simulink model "group_2_4081_4102_4209_"  (R2020a)
settings: Solver=ode23t  StartTime=0.0  StopTime=10  RelTol=1e-3
undefined symbols (not defined in the file): Acid, Lead, sigbuilder_block
libraries: powerlib x49, simulink x7, powerlib_meascontrol x5, electricdrivelib x1, re_lib x1
settings Model: Creator=ASUS  LastModifiedBy=Mushrif
settings DataIOCC: SaveOutput=off  SaveState=on  SignalLogging=off  DSMLogging=off  ReturnWorkspaceOutputs=off  LoggingToFile=on
settings DebuggingCC: UnconnectedInputMsg=none  UnconnectedOutputMsg=none  UnconnectedLineMsg=none  SFMachineParentedDataDiag=error
settings ModelReferenceCC: EnableRefExpFcnMdlSchedulingChecks=off
settings RTWCC: Description=Generic Real-Time Target

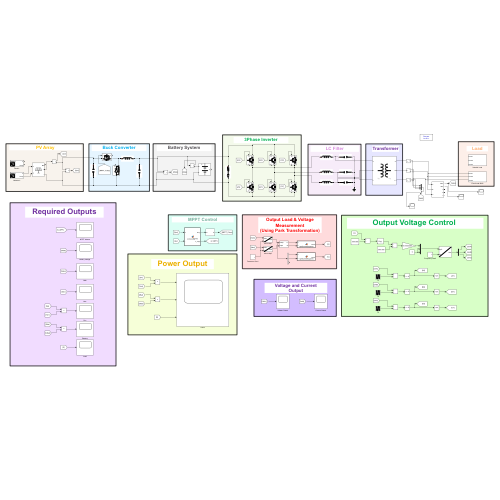
[thumbnail: Simulink's stored preview of the top-level diagram]
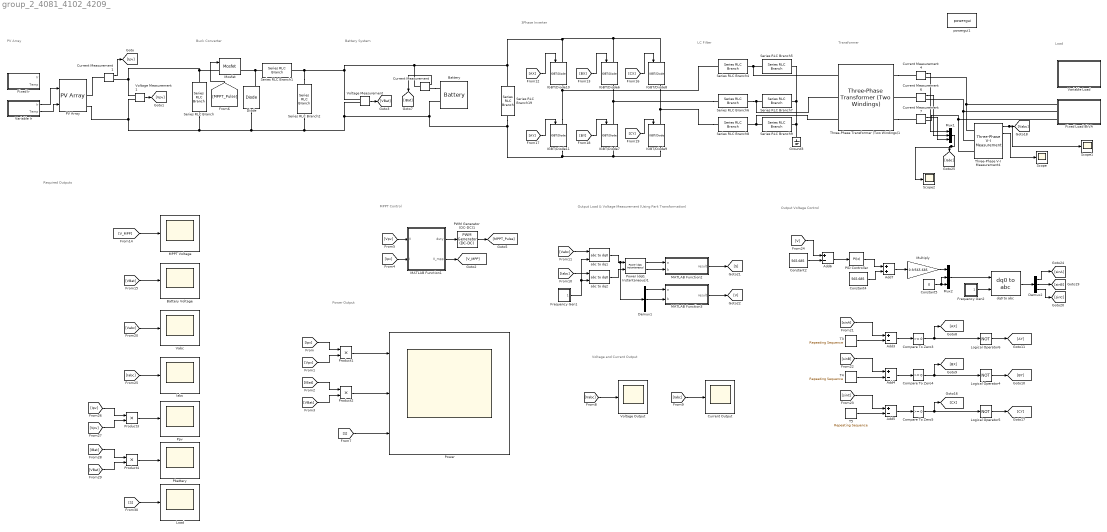
== system group_2_4081_4102_4209_ ==
  note: PV Array
  note: Buck Converter
  note: Battery System
  note: 3Phase Inverter
  note: LC Filter
  note: Load
  note: Transformer
  note: MPPT Control
  note: Power Output
  note: Output Load & Voltage Measurement
      | (Using Park Transformation)
  note: Output Voltage Control
  note: Voltage and Current
      | Output
  note: Required Outputs
  Add{3..6} (4 alike) : Sum  Inputs=+-
  Add7 : Sum
  Battery : electricdrivelib/Extra Sources/Battery  BatType=Lead-Acid  ShowTempParam=off  ThermalPreset=no  ShowAgeParam=off  NomV=48  NomQ=833.33  SOC=50  Batt_Tr=1  PresetModel=off  MaxQ=5.4  MinV=36  FullV=48  Dis_rate=2.3478  R=0.013333  Normal_OP=4.8835  expZone="[48     0.2653]"  current=[6.5 13 32.5]  Units=Time  Tci=20  NomT=20  T2=-30  MaxQ2=4.8  FullV2=7.1  Normal_OP2=5.655  expZone2="[6.58           1]"  Rca=0.6  ti=2000  Dp=0  Neq0=0  Tsim=1e6  Ta1=25  Qeol=5.4*0.9  Reol=0.013333*1.2  Char_age=[2.3478, 3]  Dis_age=[2.3478, 10]  N1=1500  N2=10500  N3=1000  N4=1400  Ta2=45  N5=950
  Battery Voltage : Scope
  Compare To Zero3 : simulink/Logic and Bit Operations/Compare To Zero  relop=>=  OutDataTypeStr=boolean
  Compare To Zero4 : simulink/Logic and Bit Operations/Compare To Zero  relop=>=  OutDataTypeStr=boolean
  Compare To Zero5 : simulink/Logic and Bit Operations/Compare To Zero  relop=>=  OutDataTypeStr=boolean
  Constant2 : Constant  Value=565.685
  Constant4 : Constant  Value=565.685
  Constant5 : Constant  Value=0
  Current Measurement{,1,4,6..7} (5 alike) : powerlib/Measurements/Current Measurement  PhasorSimulation=off  OutputType=Complex  PSBequivalent=0
  Current Output : Scope
  Demux1 : Demux  Outputs=3
  Demux2 : Demux  Outputs=3
  Diode : powerlib/Power Electronics/Diode  Ron=0.001  Lon=0  Vf=0.8  IC=0  UseSnubber=0  Rs=500  Cs=250e-9  Measurements=on
  Fixed Ir : Subsystem  Tag=STV Subsys  LoadFcn=sigbuilder_block('load');  StartFcn=sigbuilder_block('start');  StopFcn=sigbuilder_block('stop');  ClipboardFcn=sigbuilder_block('clipboard');  mask(Sigbuilder block){tuvar=[0:10]}
      mask help: Simulink:masks:SigbuilderBlock_MD
      mask init:
      | if ~strcmp(get_param(bdroot(gcbh),'SimulationStatus'),'stopped') tuvar = sigbuilder_block('maskInit'); end
      settings: CopyFcn=sigbuilder_block('copy');  DeleteFcn=sigbuilder_block('delete');  ModelCloseFcn=sigbuilder_block('modelClose');  PreSaveFcn=sigbuilder_block('preSave');  PauseFcn=sigbuilder_block('pause');  ContinueFcn=sigbuilder_block('continue');  NameChangeFcn=sigbuilder_block('namechange');  OpenFcn=sigbuilder_block('open',[437.6 182.4 550.4 400.2 ]);  CloseFcn=sigbuilder_block('close');
      mask Display: plot(0, 0, 100, 100,[2, 2, 32, 32, 2], [68, 8, 8, 68, 68],[32, 2], [38, 38], [32, 19, 2],[53, 60, 44], [32, 17, 17, 2],[16, 16, 31, 31]);txt = getActiveGroup(gcbh);text(2, 100, txt,'verticalAlignment', 'top');
  Fixed Load 8kVA : Subsystem
  Frequency Gen1 : Subsystem
  Frequency Gen2 : Subsystem
  Ground3 : powerlib/Elements/Ground  LConnTagsString=a
  IGBT/Diode{6..11} (6 alike) : powerlib/Power Electronics/IGBT//Diode  Ron=1e-3  Rs=1e5  Cs=inf  Measurements=on
  Iabc : Scope
  Load : Scope
  Logical Operator4 : Logic  Operator=NOT  AllPortsSameDT=off  OutDataTypeStr=boolean
  Logical Operator5 : Logic  Operator=NOT  AllPortsSameDT=off  OutDataTypeStr=boolean
  Logical Operator6 : Logic  Operator=NOT  AllPortsSameDT=off  OutDataTypeStr=boolean
  MATLAB Function1 : MATLAB Function  TreatAsAtomicUnit=on
  MATLAB Function2 : MATLAB Function  TreatAsAtomicUnit=on
  MATLAB Function3 : MATLAB Function  TreatAsAtomicUnit=on
  MPPT Voltage : Scope
  Mosfet : powerlib/Power Electronics/Mosfet  Ron=0.1  Lon=0  Rd=0.01  Vfd=0  IC=0  Rs=1e5  Cs=inf  Measurements=on
  Multiply : Gain  Gain=0.9/565.685
  Mux1 : Mux  Inputs=3
  Mux2 : Mux  Inputs=3
  PID Controller : simulink/Continuous/PID Controller  Controller=PI  Form=Parallel  TimeDomain=Discrete-time  UseExternalTs=off  SampleTime=-1  IntegratorMethod=Forward Euler  ControllerParametersSource=internal  P=1  I=20  D=0  N=100  UseFilter=on  TunerSelectOption=Transfer Function Based (PID Tuner App)  InitialConditionSource=internal  InitialConditionForIntegrator=0  InitialConditionForFilter=0  DifferentiatorICPrevScaledInput=0  ExternalReset=none  TrackingMode=off  Kt=1  LimitOutput=off  UpperSaturationLimit=inf  LowerSaturationLimit=-inf  LinearizeAsGain=on  AntiWindupMode=none  Kb=1  POutMin=[]  POutMax=[]  IOutMin=[]  IOutMax=[]  DOutMin=[]  DOutMax=[]  NOutMin=[]  NOutMax=[]  SumOutMin=[]  SumOutMax=[]  SaturationOutMin=[]  SaturationOutMax=[]  PParamMin=[]  PParamMax=[]  IParamMin=[]  IParamMax=[]  DParamMin=[]  DParamMax=[]  NParamMin=[]  NParamMax=[]  KbParamMin=[]  KbParamMax=[]  KtParamMin=[]  KtParamMax=[]  KbOutMin=[]  KbOutMax=[]  KtOutMin=[]  KtOutMax=[]  IntegratorOutMin=[]  IntegratorOutMax=[]  FilterOutMin=[]  FilterOutMax=[]  SumI1OutMin=[]  SumI1OutMax=[]  SumI2OutMin=[]  SumI2OutMax=[]  SumI3OutMin=[]  SumI3OutMax=[]  SumI4OutMin=[]  SumI4OutMax=[]  SumDOutMin=[]  SumDOutMax=[]  DifferentiatorOutMin=[]  DifferentiatorOutMax=[]  FilterDiffOutCoefMin=[]  FilterDiffOutCoefMax=[]  ReciprocalOutMin=[]  ReciprocalOutMax=[]  SumDenOutMin=[]  SumDenOutMax=[]  SumNumOutMin=[]  SumNumOutMax=[]  DivideOutMin=[]  DivideOutMax=[]  UdiffTsProdOutMin=[]  UdiffTsProdOutMax=[]  NTsProdOutMin=[]  NTsProdOutMax=[]  UintegralTsProdOutMin=[]  UintegralTsProdOutMax=[]  UngainTsProdOutMin=[]  UngainTsProdOutMax=[]  IntegratorContinuousStateAttributes=''  IntegratorStateMustResolveToSignalObject=off  IntegratorRTWStateStorageClass=Auto  FilterContinuousStateAttributes=''  FilterStateMustResolveToSignalObject=off  FilterRTWStateStorageClass=Auto  ParallelPVariant=InternalParameters  IdealPVariant=Disabled  IVariant=InternalParameters  DVariant=Disabled  IntegratorVariant=Discrete  SatVariant=Disabled  AWVariant=Passthrough  PCopyVariant=Disabled  TRVariant=Disabled  FdbkBlocksVariant=Forward  IdealPFdbkVariant=Disabled  SatFdbkVariant=Disabled  DerivativeFilterVariant=Disabled  NVariant=Disabled  NCopyVariant=Disabled_SignalSpec  FilterICVariant=Disabled  IntegratorICVariant=InternalICs  ExternalResetVariant=Disabled  TRSumVariant=Passthrough  SumFdbkVariant=Disabled  SumVariant=Sum_PI  TsampFilterVariant=InternalTs  TsampNgainVariant=Passthrough  TsampIntegralVariant=Passthrough
  PV Array : re_lib/Solar/PV Array  Npar=9  Nser=6  PlotType=array @ 25 deg.C & specified irradiances  S_vec="[ 1000  500  100 ]"  Temp_C_vec="[ 45 25  ]"  ModuleName=SunPower SPR-230NE-BLK-D  PlotWhenSelected=off  Pm=230.04  Ncell=72  Voc=48.2  Isc=6.05  Vm=40.5  Im=5.68  beta_Voc_pc=-0.252  alpha_Isc_pc=0.039008  beta_Voc=-0.12146  alpha_Isc=0.00236  IL=6.0576  I0=2.3299e-12  nI=0.91228  Rsh=325.3067  Rs=0.4111  RobustModel=off  RobustCellTemperature=25  BAL=on  Tc=1e-6  Tfilter=5e-5
  PWM Generator (DC-DC)1 : powerlib_meascontrol/Pulse & Signal Generators/PWM Generator (DC-DC)  Fsw=20000  Ts=1e-6
  Pbattery : Scope
  Power : Scope  NumInputPorts=3
  "Power (dq0, Instantaneous)1" : powerlib_meascontrol/Measurements/Power (dq0, Instantaneous)
      link override pu->V2: Gain=0.86486
      link override pu->V3: Gain=0.86486
  Ppv : Scope
  Product{1..4} (4 alike) : Product
  Scope : Scope
  Scope1 : Scope
  Scope2 : Scope
  Series RLC Branch : powerlib/Elements/Series RLC Branch  LConnTagsString=__new0  RConnTagsString=__new0  BranchType=C  Resistance=0.0001  Inductance=1e-3  SetiL0=off  InitialCurrent=0  Capacitance=40e-3  Setx0=off  InitialVoltage=0  Measurements=None
  Series RLC Branch1 : powerlib/Elements/Series RLC Branch  LConnTagsString=__new0  RConnTagsString=__new0  BranchType=L  Resistance=1  Inductance=250e-3  SetiL0=off  InitialCurrent=0  Capacitance=1e-6  Setx0=off  InitialVoltage=0  Measurements=None
  Series RLC Branch19 : powerlib/Elements/Series RLC Branch  LConnTagsString=__new0  RConnTagsString=__new0  BranchType=RC  Resistance=0.02  Inductance=1e-3  SetiL0=off  InitialCurrent=0  Capacitance=0.001  Setx0=off  InitialVoltage=0  Measurements=None
  Series RLC Branch2 : powerlib/Elements/Series RLC Branch  LConnTagsString=__new0  RConnTagsString=__new0  BranchType=C  Resistance=1  Inductance=0.0474  SetiL0=off  InitialCurrent=0  Capacitance=100e-3  Setx0=off  InitialVoltage=0  Measurements=None
  Series RLC Branch4 : powerlib/Elements/Series RLC Branch  LConnTagsString=__new0  RConnTagsString=__new0  BranchType=L  Resistance=2.2  Inductance=250e-6  SetiL0=off  InitialCurrent=0  Capacitance=1e-6  Setx0=off  InitialVoltage=0  Measurements=None
  Series RLC Branch5 : powerlib/Elements/Series RLC Branch  LConnTagsString=__new0  RConnTagsString=__new0  BranchType=C  Resistance=1  Inductance=1e-3  SetiL0=off  InitialCurrent=0  Capacitance=40e-6  Setx0=off  InitialVoltage=0  Measurements=None
  Series RLC Branch6 : powerlib/Elements/Series RLC Branch  LConnTagsString=__new0  RConnTagsString=__new0  BranchType=L  Resistance=2.2  Inductance=250e-6  SetiL0=off  InitialCurrent=0  Capacitance=1e-6  Setx0=off  InitialVoltage=0  Measurements=None
  Series RLC Branch7 : powerlib/Elements/Series RLC Branch  LConnTagsString=__new0  RConnTagsString=__new0  BranchType=C  Resistance=1  Inductance=1e-3  SetiL0=off  InitialCurrent=0  Capacitance=40e-6  Setx0=off  InitialVoltage=0  Measurements=None
  Series RLC Branch8 : powerlib/Elements/Series RLC Branch  LConnTagsString=__new0  RConnTagsString=__new0  BranchType=L  Resistance=2.2  Inductance=250e-6  SetiL0=off  InitialCurrent=0  Capacitance=1e-6  Setx0=off  InitialVoltage=0  Measurements=None
  Series RLC Branch9 : powerlib/Elements/Series RLC Branch  LConnTagsString=__new0  RConnTagsString=__new0  BranchType=C  Resistance=1  Inductance=1e-3  SetiL0=off  InitialCurrent=0  Capacitance=40e-6  Setx0=off  InitialVoltage=0  Measurements=None
  T3 : simulink/Sources/Repeating Sequence  rep_seq_t=[0 0.0000125 0.000025 0.0000375 0.00005]  rep_seq_y=[0 -1 0 1 0]
  T4 : simulink/Sources/Repeating Sequence  rep_seq_t=[0 0.0000125 0.000025 0.0000375 0.00005]  rep_seq_y=[0 -1 0 1 0]
  T5 : simulink/Sources/Repeating Sequence  rep_seq_t=[0 0.0000125 0.000025 0.0000375 0.00005]  rep_seq_y=[0 -1 0 1 0]
  Three-Phase Transformer (Two Windings)1 : powerlib/Elements/Three-Phase Transformer (Two Windings)  Winding1Connection=Yg  Winding2Connection=Yg  CoreType=Three single-phase transformers  SetSaturation=off  Hysteresis=off  DataFile='hysteresis'  SetInitialFlux=off  Measurements=None  UNITS=SI  NominalPower=[ 8000 , 50 ]  Winding1=[400 0.000001 0.00000000001]  Winding2=[25 0.000001 0.00000000001]  Rm=10000000000  Lm=1000  L0=0.5  Saturation=[0 0;0.0089716 1.2943;3.7382 1.6394]  InitialFluxes=[ 0.8 , -0.8 , 0.7 ]  BreakLoop=off  DiscreteSolver=Trapezoidal iterative  DataType=on  TransfoNumber=1
  Three-Phase V-I Measurement4 : powerlib/Measurements/Three-Phase V-I Measurement  VoltageMeasurement=phase-to-phase  SetLabelV=off  LabelV=Vabc  Vpu=off  VpuLL=off  CurrentMeasurement=yes  SetLabelI=off  LabelI=Iabc  Ipu=off  Pbase=100e6  Vbase=500e3  OutputType=Complex  PhasorSimulation=off  PSBequivalent=0
  Vabc : Scope
  Variable Ir : Subsystem  Tag=STV Subsys  LoadFcn=sigbuilder_block('load');  StartFcn=sigbuilder_block('start');  StopFcn=sigbuilder_block('stop');  ClipboardFcn=sigbuilder_block('clipboard');  mask(Sigbuilder block){tuvar=[0:10]}
      mask help: Simulink:masks:SigbuilderBlock_MD
      mask init:
      | if ~strcmp(get_param(bdroot(gcbh),'SimulationStatus'),'stopped') tuvar = sigbuilder_block('maskInit'); end
      settings: CopyFcn=sigbuilder_block('copy');  DeleteFcn=sigbuilder_block('delete');  ModelCloseFcn=sigbuilder_block('modelClose');  PreSaveFcn=sigbuilder_block('preSave');  PauseFcn=sigbuilder_block('pause');  ContinueFcn=sigbuilder_block('continue');  NameChangeFcn=sigbuilder_block('namechange');  OpenFcn=sigbuilder_block('open',[437.6 182.4 550.4 400.2 ]);  CloseFcn=sigbuilder_block('close');
      mask Display: plot(0, 0, 100, 100,[2, 2, 32, 32, 2], [68, 8, 8, 68, 68],[32, 2], [38, 38], [32, 19, 2],[53, 60, 44], [32, 17, 17, 2],[16, 16, 31, 31]);txt = getActiveGroup(gcbh);text(2, 100, txt,'verticalAlignment', 'top');
  Variable Load : Subsystem
  Voltage Measurement : powerlib/Measurements/Voltage Measurement  PhasorSimulation=off  OutputType=Complex  PSBequivalent=0
  Voltage Measurement1 : powerlib/Measurements/Voltage Measurement  PhasorSimulation=off  OutputType=Complex  PSBequivalent=0
  Voltage Output : Scope
  abc to dq1 : powerlib_meascontrol/Transformations/abc to dq0  Alignment=Aligned with phase A axis
  abc to dq2 : powerlib_meascontrol/Transformations/abc to dq0  Alignment=Aligned with phase A axis
  dq0 to abc : powerlib_meascontrol/Transformations/dq0 to abc  Alignment=90 degrees behind phase A axis
  powergui1 : powerlib/powergui  Priority=1  SimulationMode=Discrete  SampleTime=1e-6  frequency=60  Iterations=50  frequencyindice=0  Pbase=100e6  ErrMax=1e-4  UnitsV=kV  UnitsW=MW  buscounter=0  FunctionMessages=off  echomessages=off  EnableUseOfTLC=off  CurrentSourceSwitches=off  DisableSnubberDevices=off  DisableRonSwitches=off  DisableVfSwitches=off  DisplayEquations=off  AutomaticDiscreteSolvers=off  SolverType=Tustin/Backward Euler (TBE)  Interpol=off  ExternalGateDelay=off  methode=off  Ts=100  x0status=blocks  SPID=on  SwTol=0  HookPort=off  NonlinearTolerance=1e-4  nMaxIteration=100  ContinueOnMaxIteration=off  RestoreLinks=warning  ResistiveCurrentMeasurement=off  Frange=[0:2:500]  Ylog=off  Xlog=on  ShowGrid=off  save=off  variable=ZData  structure=0  ZoomFFT=off  StartTime=0.0  cycles=1  DisplayStyle=1  fundamental=60  FreqAxis=off  MaxFrequency=1000  frequencyindicesteady=1  RmsSteady=1  display=off
  wires:
  Voltage Measurement/1 -> [VBat]
  Current Measurement1/1 -> [Ipv]
  Voltage Measurement1/1 -> [Vpv]
  [Ipv] -> Product1/1
  [Vpv] -> Product1/2
  Product1/1 -> Power/1
  PWM Generator (DC-DC)1/1 -> [MPPT_Pulse]
  MATLAB Function1/1(duty) -> PWM Generator (DC-DC)1/1
  [Vpv] -> MATLAB Function1/1(V)
  [Ipv] -> MATLAB Function1/2(I)
  [MPPT_Pulse] -> Mosfet/1
  Constant4/1 -> Add7/2
  dq0 to abc/1 -> Demux2/1
  Demux2/3 -> [sinC]
  PID Controller/1 -> Add7/1
  Demux1/2 -> MATLAB Function3/2(b)
  Multiply/1 -> Mux2/1
  "Power (dq0, Instantaneous)1"/1 -> MATLAB Function2/1(a)
  [BX] -> IGBT/Diode6/1
  [AY] -> IGBT/Diode11/1
  Mux1/1 -> Scope2/1, [Iabc]
  Constant5/1 -> Mux2/3, Mux2/2
  Mux2/1 -> dq0 to abc/1
  Demux1/1 -> MATLAB Function3/1(a)
  [AX] -> IGBT/Diode10/1
  Three-Phase V-I Measurement4/1 -> Scope1/1, [Vabc]
  Current Measurement4/1 -> Mux1/1
  [BY] -> IGBT/Diode7/1
  Current Measurement6/1 -> Mux1/2
  Constant2/1 -> Add6/2
  [CY] -> IGBT/Diode9/1
  Frequency Gen2/1(Out1) -> dq0 to abc/2
  MATLAB Function2/1(result) -> [S]
  Current Measurement7/1 -> Mux1/3
  Demux2/2 -> [sinB]
  Add6/1 -> PID Controller/1
  Add7/1 -> Multiply/1
  [Iabc] -> abc to dq2/1
  MATLAB Function3/1(result) -> [V]
  "Power (dq0, Instantaneous)1"/2 -> MATLAB Function2/2(b)
  Demux2/1 -> [sinA]
  [CX] -> IGBT/Diode8/1
  [IBat] -> Product2/1
  [VBat] -> Product2/2
  Product2/1 -> Power/2
  [S] -> Power/3
  [V] -> Add6/1
  Current Measurement/1 -> [IBat]
  abc to dq2/1 -> "Power (dq0, Instantaneous)1"/2
  abc to dq1/1 -> "Power (dq0, Instantaneous)1"/1, Demux1/1
  [Vabc] -> abc to dq1/1
  Frequency Gen1/1(Out1) -> abc to dq1/2, abc to dq2/2
  Three-Phase V-I Measurement4/2 -> Scope/1
  [sinA] -> Add3/1
  Add5/1 -> Compare To Zero5/1
  Compare To Zero3/1 -> Logical Operator6/1, [AX]
  Logical Operator6/1 -> [AY]
  T5/1 -> Add5/2
  Compare To Zero4/1 -> Logical Operator4/1, [BX]
  Add3/1 -> Compare To Zero3/1
  T3/1 -> Add3/2
  Logical Operator4/1 -> [BY]
  [sinB] -> Add4/1
  Compare To Zero5/1 -> Logical Operator5/1, [CX]
  T4/1 -> Add4/2
  Logical Operator5/1 -> [CY]
  Add4/1 -> Compare To Zero4/1
  [sinC] -> Add5/1
  [Vabc] -> Voltage Output/1
  [Iabc] -> Current Output/1
  [V_MPP] -> MPPT Voltage/1
  [VBat] -> Battery Voltage/1
  [Vabc] -> Vabc/1
  [Iabc] -> Iabc/1
  [Vpv] -> Product3/2
  [Ipv] -> Product3/1
  Product3/1 -> Ppv/1
  [IBat] -> Product4/1
  [VBat] -> Product4/2
  Product4/1 -> Pbattery/1
  [S] -> Load/1
  MATLAB Function1/2(V_mpp) -> [V_MPP]
  Variable Ir/1(Ir) -> PV Array/1
  Variable Ir/2(Temp) -> PV Array/2
  connections:
  Mosfet/LConn1 -- Voltage Measurement1/LConn1 -- Current Measurement1/RConn1 -- Series RLC Branch/LConn1
  Diode/RConn1 -- Mosfet/RConn1 -- Series RLC Branch1/LConn1
  Current Measurement1/LConn1 -- PV Array/RConn1
  Voltage Measurement1/LConn2 -- Series RLC Branch19/RConn1 -- IGBT/Diode11/RConn1 -- IGBT/Diode9/RConn1 -- IGBT/Diode7/RConn1 -- Battery/LConn2 -- Voltage Measurement/LConn2 -- Series RLC Branch2/RConn1 -- Diode/LConn1 -- Series RLC Branch/RConn1 -- PV Array/RConn2
  Series RLC Branch4/RConn1 -- Three-Phase Transformer (Two Windings)1/RConn1 -- Series RLC Branch5/LConn1
  Series RLC Branch6/LConn1 -- IGBT/Diode6/RConn1 -- IGBT/Diode7/LConn1
  Series RLC Branch8/RConn1 -- Three-Phase Transformer (Two Windings)1/RConn3 -- Series RLC Branch9/LConn1
  Three-Phase V-I Measurement4/LConn1 -- Current Measurement4/RConn1 -- Fixed Load 8kVA/LConn1
  Series RLC Branch6/RConn1 -- Three-Phase Transformer (Two Windings)1/RConn2 -- Series RLC Branch7/LConn1
  IGBT/Diode11/LConn1 -- IGBT/Diode10/RConn1 -- Series RLC Branch4/LConn1
  Series RLC Branch5/RConn1 -- Series RLC Branch7/RConn1 -- Ground3/LConn1 -- Series RLC Branch9/RConn1
  Three-Phase V-I Measurement4/LConn3 -- Fixed Load 8kVA/LConn3 -- Current Measurement7/RConn1
  Series RLC Branch8/LConn1 -- IGBT/Diode8/RConn1 -- IGBT/Diode9/LConn1
  Three-Phase V-I Measurement4/LConn2 -- Fixed Load 8kVA/LConn2 -- Current Measurement6/RConn1
  Three-Phase Transformer (Two Windings)1/LConn3 -- Current Measurement7/LConn1
  Three-Phase Transformer (Two Windings)1/LConn1 -- Current Measurement4/LConn1
  Current Measurement6/LConn1 -- Three-Phase Transformer (Two Windings)1/LConn2
  Series RLC Branch2/LConn1 -- IGBT/Diode8/LConn1 -- IGBT/Diode6/LConn1 -- IGBT/Diode10/LConn1 -- Series RLC Branch19/LConn1 -- Current Measurement/LConn1 -- Voltage Measurement/LConn1 -- Series RLC Branch1/RConn1
  Current Measurement/RConn1 -- Battery/LConn1

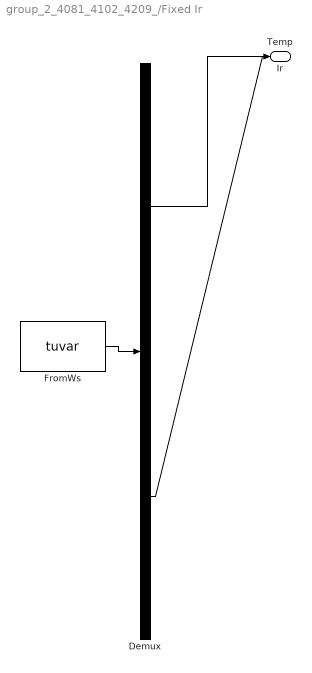
== system group_2_4081_4102_4209_/Fixed Ir ==
  Demux : Demux  Tag=STV Demux  Outputs=2
      settings: DisplayOption=none
  FromWs : FromWorkspace  Tag=STV FromWs  VariableName=tuvar
      SigBuilderData=|
      | common.afterFinalStr = 'Extrapolate'
      | common.sampleTime = 0
      | dataSet.timeRange = [0 10]
      | dataSet.name = 'Group 1'
      | sbobj.Groups.Name = 'Group 1'
      | sbobj.Groups.Signals(1).Name = 'Ir'
      | sbobj.Groups.Signals(1).XData = [0 5 8 10]
      | sbobj.Groups.Signals(1).YData = [1000 1000 1000 1000]
      | sbobj.Groups.Signals(2).Name = 'Temp'
      | sbobj.Groups.Signals(2).XData = [0 4 6 10]
      | sbobj.Groups.Signals(2).YData = [25 25 25 25]
  Ir : Outport  Tag=STV Outport
  Temp : Outport  Tag=STV Outport  Port=2
  wires:
  FromWs/1 -> Demux/1
  Demux/1 -> Ir/1
  Demux/2 -> Temp/1

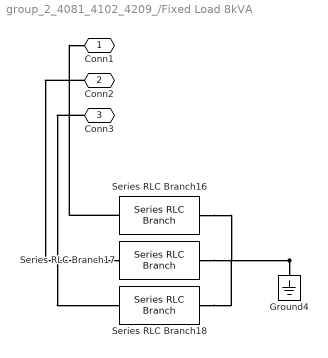
== system group_2_4081_4102_4209_/Fixed Load 8kVA ==
  Ground4 : powerlib/Elements/Ground  LConnTagsString=a
  Series RLC Branch16 : powerlib/Elements/Series RLC Branch  LConnTagsString=__new0  RConnTagsString=__new0  BranchType=R  Resistance=20  Inductance=1e-3  SetiL0=off  InitialCurrent=0  Capacitance=1e-6  Setx0=off  InitialVoltage=0  Measurements=None
  Series RLC Branch17 : powerlib/Elements/Series RLC Branch  LConnTagsString=__new0  RConnTagsString=__new0  BranchType=R  Resistance=20  Inductance=1e-3  SetiL0=off  InitialCurrent=0  Capacitance=1e-6  Setx0=off  InitialVoltage=0  Measurements=None
  Series RLC Branch18 : powerlib/Elements/Series RLC Branch  LConnTagsString=__new0  RConnTagsString=__new0  BranchType=R  Resistance=20  Inductance=1e-3  SetiL0=off  InitialCurrent=0  Capacitance=1e-6  Setx0=off  InitialVoltage=0  Measurements=None
  Conn1 : PMIOPort  Side=Left
  Conn2 : PMIOPort  Port=2  Side=Left
  Conn3 : PMIOPort  Port=3  Side=Left
  connections:
  Conn3/RConn1 -- Series RLC Branch18/LConn1
  Ground4/LConn1 -- Series RLC Branch16/RConn1 -- Series RLC Branch18/RConn1 -- Series RLC Branch17/RConn1
  Conn2/RConn1 -- Series RLC Branch17/LConn1
  Series RLC Branch16/LConn1 -- Conn1/RConn1

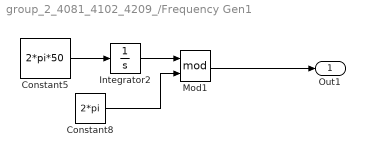
== system group_2_4081_4102_4209_/Frequency Gen1 ==
  Constant5 : Constant  Value=2*pi*50
  Constant8 : Constant  Value=2*pi
  Integrator2 : Integrator
  Mod1 : Math  Operator=mod  SaturateOnIntegerOverflow=on
  Out1 : Outport
  wires:
  Mod1/1 -> Out1/1
  Constant5/1 -> Integrator2/1
  Constant8/1 -> Mod1/2
  Integrator2/1 -> Mod1/1

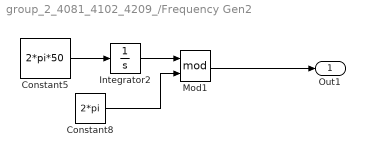
== system group_2_4081_4102_4209_/Frequency Gen2 ==
  Constant5 : Constant  Value=2*pi*50
  Constant8 : Constant  Value=2*pi
  Integrator2 : Integrator
  Mod1 : Math  Operator=mod  SaturateOnIntegerOverflow=on
  Out1 : Outport
  wires:
  Mod1/1 -> Out1/1
  Constant5/1 -> Integrator2/1
  Constant8/1 -> Mod1/2
  Integrator2/1 -> Mod1/1

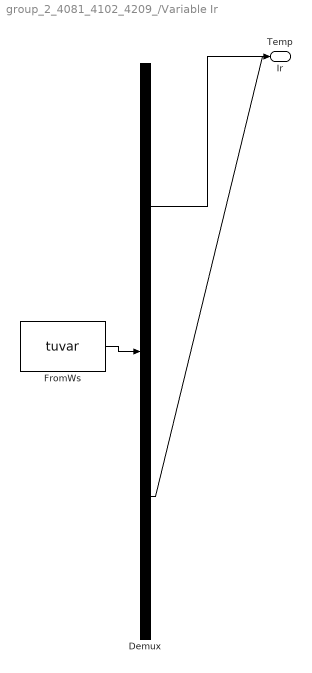
== system group_2_4081_4102_4209_/Variable Ir ==
  Demux : Demux  Tag=STV Demux  Outputs=2
      settings: DisplayOption=none
  FromWs : FromWorkspace  Tag=STV FromWs  VariableName=tuvar
      SigBuilderData=|
      | common.afterFinalStr = 'Extrapolate'
      | common.sampleTime = 0
      | dataSet.timeRange = [0 10]
      | dataSet.name = 'Group 1'
      | sbobj.Groups.Name = 'Group 1'
      | sbobj.Groups.Signals(1).Name = 'Ir'
      | sbobj.Groups.Signals(1).XData = [0 5 5 8 8 10]
      | sbobj.Groups.Signals(1).YData = [500 500 1000 1000 700 700]
      | sbobj.Groups.Signals(2).Name = 'Temp'
      | sbobj.Groups.Signals(2).XData = [0 4 6 10]
      | sbobj.Groups.Signals(2).YData = [25 25 25 25]
  Ir : Outport  Tag=STV Outport
  Temp : Outport  Tag=STV Outport  Port=2
  wires:
  FromWs/1 -> Demux/1
  Demux/1 -> Ir/1
  Demux/2 -> Temp/1

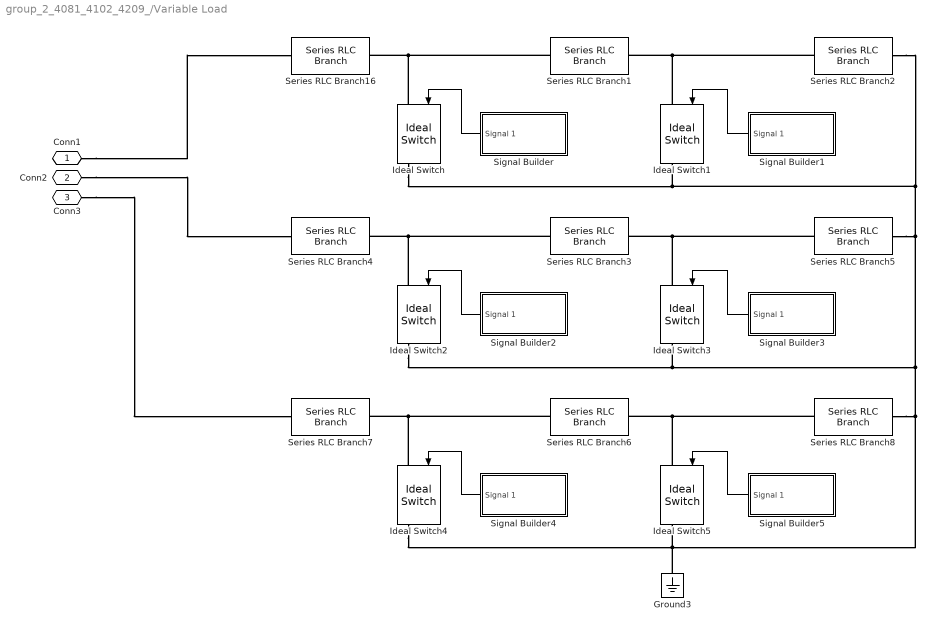
== system group_2_4081_4102_4209_/Variable Load ==
  Ground3 : powerlib/Elements/Ground  LConnTagsString=a
  Ideal Switch{,1..5} (6 alike) : powerlib/Power Electronics/Ideal Switch  Ron=0.001  Lon=0  IC=0  Rs=1e5  Cs=inf  Measurements=on
  Series RLC Branch1 : powerlib/Elements/Series RLC Branch  LConnTagsString=__new0  RConnTagsString=__new0  BranchType=R  Resistance=13.33  Inductance=1e-3  SetiL0=off  InitialCurrent=0  Capacitance=1e-6  Setx0=off  InitialVoltage=0  Measurements=None
  Series RLC Branch16 : powerlib/Elements/Series RLC Branch  LConnTagsString=__new0  RConnTagsString=__new0  BranchType=R  Resistance=20  Inductance=1e-3  SetiL0=off  InitialCurrent=0  Capacitance=1e-6  Setx0=off  InitialVoltage=0  Measurements=None
  Series RLC Branch2 : powerlib/Elements/Series RLC Branch  LConnTagsString=__new0  RConnTagsString=__new0  BranchType=R  Resistance=6.67  Inductance=1e-3  SetiL0=off  InitialCurrent=0  Capacitance=1e-6  Setx0=off  InitialVoltage=0  Measurements=None
  Series RLC Branch3 : powerlib/Elements/Series RLC Branch  LConnTagsString=__new0  RConnTagsString=__new0  BranchType=R  Resistance=13.33  Inductance=1e-3  SetiL0=off  InitialCurrent=0  Capacitance=1e-6  Setx0=off  InitialVoltage=0  Measurements=None
  Series RLC Branch4 : powerlib/Elements/Series RLC Branch  LConnTagsString=__new0  RConnTagsString=__new0  BranchType=R  Resistance=20  Inductance=1e-3  SetiL0=off  InitialCurrent=0  Capacitance=1e-6  Setx0=off  InitialVoltage=0  Measurements=None
  Series RLC Branch5 : powerlib/Elements/Series RLC Branch  LConnTagsString=__new0  RConnTagsString=__new0  BranchType=R  Resistance=6.67  Inductance=1e-3  SetiL0=off  InitialCurrent=0  Capacitance=1e-6  Setx0=off  InitialVoltage=0  Measurements=None
  Series RLC Branch6 : powerlib/Elements/Series RLC Branch  LConnTagsString=__new0  RConnTagsString=__new0  BranchType=R  Resistance=13.33  Inductance=1e-3  SetiL0=off  InitialCurrent=0  Capacitance=1e-6  Setx0=off  InitialVoltage=0  Measurements=None
  Series RLC Branch7 : powerlib/Elements/Series RLC Branch  LConnTagsString=__new0  RConnTagsString=__new0  BranchType=R  Resistance=20  Inductance=1e-3  SetiL0=off  InitialCurrent=0  Capacitance=1e-6  Setx0=off  InitialVoltage=0  Measurements=None
  Series RLC Branch8 : powerlib/Elements/Series RLC Branch  LConnTagsString=__new0  RConnTagsString=__new0  BranchType=R  Resistance=6.67  Inductance=1e-3  SetiL0=off  InitialCurrent=0  Capacitance=1e-6  Setx0=off  InitialVoltage=0  Measurements=None
  Signal Builder : Subsystem  Tag=STV Subsys  LoadFcn=sigbuilder_block('load');  StartFcn=sigbuilder_block('start');  StopFcn=sigbuilder_block('stop');  ClipboardFcn=sigbuilder_block('clipboard');  mask(Sigbuilder block){tuvar=[0:10]}
      mask help: Simulink:masks:SigbuilderBlock_MD
      mask init:
      | if ~strcmp(get_param(bdroot(gcbh),'SimulationStatus'),'stopped') tuvar = sigbuilder_block('maskInit'); end
      settings: CopyFcn=sigbuilder_block('copy');  DeleteFcn=sigbuilder_block('delete');  ModelCloseFcn=sigbuilder_block('modelClose');  PreSaveFcn=sigbuilder_block('preSave');  PauseFcn=sigbuilder_block('pause');  ContinueFcn=sigbuilder_block('continue');  NameChangeFcn=sigbuilder_block('namechange');  OpenFcn=sigbuilder_block('open',[437.6 199.2 550.4 400 ]);  CloseFcn=sigbuilder_block('close');
      mask Display: plot(0, 0, 100, 100,[2, 2, 32, 32, 2], [68, 8, 8, 68, 68],[32, 2], [38, 38], [32, 19, 2],[53, 60, 44], [32, 17, 17, 2],[16, 16, 31, 31]);txt = getActiveGroup(gcbh);text(2, 100, txt,'verticalAlignment', 'top');
  Signal Builder1 : Subsystem  Tag=STV Subsys  LoadFcn=sigbuilder_block('load');  StartFcn=sigbuilder_block('start');  StopFcn=sigbuilder_block('stop');  ClipboardFcn=sigbuilder_block('clipboard');  mask(Sigbuilder block){tuvar=[0:10]}
      mask help: Simulink:masks:SigbuilderBlock_MD
      mask init:
      | if ~strcmp(get_param(bdroot(gcbh),'SimulationStatus'),'stopped') tuvar = sigbuilder_block('maskInit'); end
      settings: CopyFcn=sigbuilder_block('copy');  DeleteFcn=sigbuilder_block('delete');  ModelCloseFcn=sigbuilder_block('modelClose');  PreSaveFcn=sigbuilder_block('preSave');  PauseFcn=sigbuilder_block('pause');  ContinueFcn=sigbuilder_block('continue');  NameChangeFcn=sigbuilder_block('namechange');  OpenFcn=sigbuilder_block('open',[437.6 199.2 550.4 400 ]);  CloseFcn=sigbuilder_block('close');
      mask Display: plot(0, 0, 100, 100,[2, 2, 32, 32, 2], [68, 8, 8, 68, 68],[32, 2], [38, 38], [32, 19, 2],[53, 60, 44], [32, 17, 17, 2],[16, 16, 31, 31]);txt = getActiveGroup(gcbh);text(2, 100, txt,'verticalAlignment', 'top');
  Signal Builder2 : Subsystem  Tag=STV Subsys  LoadFcn=sigbuilder_block('load');  StartFcn=sigbuilder_block('start');  StopFcn=sigbuilder_block('stop');  ClipboardFcn=sigbuilder_block('clipboard');  mask(Sigbuilder block){tuvar=[0:10]}
      mask help: Simulink:masks:SigbuilderBlock_MD
      mask init:
      | if ~strcmp(get_param(bdroot(gcbh),'SimulationStatus'),'stopped') tuvar = sigbuilder_block('maskInit'); end
      settings: CopyFcn=sigbuilder_block('copy');  DeleteFcn=sigbuilder_block('delete');  ModelCloseFcn=sigbuilder_block('modelClose');  PreSaveFcn=sigbuilder_block('preSave');  PauseFcn=sigbuilder_block('pause');  ContinueFcn=sigbuilder_block('continue');  NameChangeFcn=sigbuilder_block('namechange');  OpenFcn=sigbuilder_block('open',[437.6 199.2 550.4 400 ]);  CloseFcn=sigbuilder_block('close');
      mask Display: plot(0, 0, 100, 100,[2, 2, 32, 32, 2], [68, 8, 8, 68, 68],[32, 2], [38, 38], [32, 19, 2],[53, 60, 44], [32, 17, 17, 2],[16, 16, 31, 31]);txt = getActiveGroup(gcbh);text(2, 100, txt,'verticalAlignment', 'top');
  Signal Builder3 : Subsystem  Tag=STV Subsys  LoadFcn=sigbuilder_block('load');  StartFcn=sigbuilder_block('start');  StopFcn=sigbuilder_block('stop');  ClipboardFcn=sigbuilder_block('clipboard');  mask(Sigbuilder block){tuvar=[0:10]}
      mask help: Simulink:masks:SigbuilderBlock_MD
      mask init:
      | if ~strcmp(get_param(bdroot(gcbh),'SimulationStatus'),'stopped') tuvar = sigbuilder_block('maskInit'); end
      settings: CopyFcn=sigbuilder_block('copy');  DeleteFcn=sigbuilder_block('delete');  ModelCloseFcn=sigbuilder_block('modelClose');  PreSaveFcn=sigbuilder_block('preSave');  PauseFcn=sigbuilder_block('pause');  ContinueFcn=sigbuilder_block('continue');  NameChangeFcn=sigbuilder_block('namechange');  OpenFcn=sigbuilder_block('open',[437.6 199.2 550.4 400 ]);  CloseFcn=sigbuilder_block('close');
      mask Display: plot(0, 0, 100, 100,[2, 2, 32, 32, 2], [68, 8, 8, 68, 68],[32, 2], [38, 38], [32, 19, 2],[53, 60, 44], [32, 17, 17, 2],[16, 16, 31, 31]);txt = getActiveGroup(gcbh);text(2, 100, txt,'verticalAlignment', 'top');
  Signal Builder4 : Subsystem  Tag=STV Subsys  LoadFcn=sigbuilder_block('load');  StartFcn=sigbuilder_block('start');  StopFcn=sigbuilder_block('stop');  ClipboardFcn=sigbuilder_block('clipboard');  mask(Sigbuilder block){tuvar=[0:10]}
      mask help: Simulink:masks:SigbuilderBlock_MD
      mask init:
      | if ~strcmp(get_param(bdroot(gcbh),'SimulationStatus'),'stopped') tuvar = sigbuilder_block('maskInit'); end
      settings: CopyFcn=sigbuilder_block('copy');  DeleteFcn=sigbuilder_block('delete');  ModelCloseFcn=sigbuilder_block('modelClose');  PreSaveFcn=sigbuilder_block('preSave');  PauseFcn=sigbuilder_block('pause');  ContinueFcn=sigbuilder_block('continue');  NameChangeFcn=sigbuilder_block('namechange');  OpenFcn=sigbuilder_block('open',[437.6 199.2 550.4 400 ]);  CloseFcn=sigbuilder_block('close');
      mask Display: plot(0, 0, 100, 100,[2, 2, 32, 32, 2], [68, 8, 8, 68, 68],[32, 2], [38, 38], [32, 19, 2],[53, 60, 44], [32, 17, 17, 2],[16, 16, 31, 31]);txt = getActiveGroup(gcbh);text(2, 100, txt,'verticalAlignment', 'top');
  Signal Builder5 : Subsystem  Tag=STV Subsys  LoadFcn=sigbuilder_block('load');  StartFcn=sigbuilder_block('start');  StopFcn=sigbuilder_block('stop');  ClipboardFcn=sigbuilder_block('clipboard');  mask(Sigbuilder block){tuvar=[0:10]}
      mask help: Simulink:masks:SigbuilderBlock_MD
      mask init:
      | if ~strcmp(get_param(bdroot(gcbh),'SimulationStatus'),'stopped') tuvar = sigbuilder_block('maskInit'); end
      settings: CopyFcn=sigbuilder_block('copy');  DeleteFcn=sigbuilder_block('delete');  ModelCloseFcn=sigbuilder_block('modelClose');  PreSaveFcn=sigbuilder_block('preSave');  PauseFcn=sigbuilder_block('pause');  ContinueFcn=sigbuilder_block('continue');  NameChangeFcn=sigbuilder_block('namechange');  OpenFcn=sigbuilder_block('open',[437.6 199.2 550.4 400 ]);  CloseFcn=sigbuilder_block('close');
      mask Display: plot(0, 0, 100, 100,[2, 2, 32, 32, 2], [68, 8, 8, 68, 68],[32, 2], [38, 38], [32, 19, 2],[53, 60, 44], [32, 17, 17, 2],[16, 16, 31, 31]);txt = getActiveGroup(gcbh);text(2, 100, txt,'verticalAlignment', 'top');
  Conn1 : PMIOPort  Side=Left
  Conn2 : PMIOPort  Port=2  Side=Left
  Conn3 : PMIOPort  Port=3  Side=Left
  wires:
  Signal Builder5/1(Signal 1) -> Ideal Switch5/1
  Signal Builder2/1(Signal 1) -> Ideal Switch2/1
  Signal Builder4/1(Signal 1) -> Ideal Switch4/1
  Signal Builder/1(Signal 1) -> Ideal Switch/1
  Signal Builder3/1(Signal 1) -> Ideal Switch3/1
  Signal Builder1/1(Signal 1) -> Ideal Switch1/1
  connections:
  Ideal Switch4/RConn1 -- Ideal Switch/RConn1 -- Ideal Switch1/RConn1 -- Series RLC Branch2/RConn1 -- Series RLC Branch5/RConn1 -- Ideal Switch3/RConn1 -- Ideal Switch2/RConn1 -- Series RLC Branch8/RConn1 -- Ideal Switch5/RConn1 -- Ground3/LConn1
  Ideal Switch5/LConn1 -- Series RLC Branch8/LConn1 -- Series RLC Branch6/RConn1
  Ideal Switch4/LConn1 -- Series RLC Branch7/RConn1 -- Series RLC Branch6/LConn1
  Ideal Switch1/LConn1 -- Series RLC Branch2/LConn1 -- Series RLC Branch1/RConn1
  Series RLC Branch1/LConn1 -- Series RLC Branch16/RConn1 -- Ideal Switch/LConn1
  Ideal Switch3/LConn1 -- Series RLC Branch5/LConn1 -- Series RLC Branch3/RConn1
  Ideal Switch2/LConn1 -- Series RLC Branch4/RConn1 -- Series RLC Branch3/LConn1
  Conn2/RConn1 -- Series RLC Branch4/LConn1
  Conn3/RConn1 -- Series RLC Branch7/LConn1
  Conn1/RConn1 -- Series RLC Branch16/LConn1

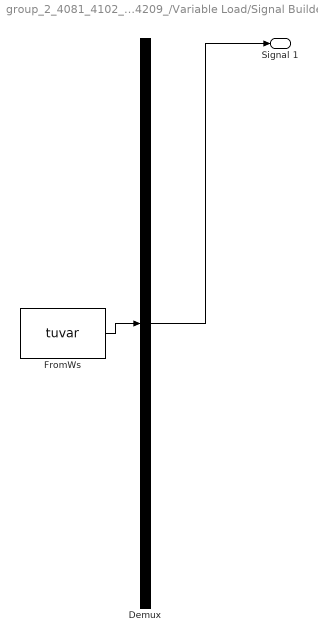
== system group_2_4081_4102_4209_/Variable Load/Signal Builder ==
  Demux : Demux  Tag=STV Demux  Outputs=1
      settings: DisplayOption=none
  FromWs : FromWorkspace  Tag=STV FromWs  VariableName=tuvar
      SigBuilderData=|
      | common.afterFinalStr = 'Extrapolate'
      | common.sampleTime = 0
      | dataSet.timeRange = [0 10]
      | dataSet.name = 'Group 1'
      | sbobj.Groups.Name = 'Group 1'
      | sbobj.Groups.Signals.Name = 'Signal 1'
      | sbobj.Groups.Signals.XData = [0 5 5 8 8 10]
      | sbobj.Groups.Signals.YData = [0 0 1 1 0 0]
  Signal 1 : Outport  Tag=STV Outport
  wires:
  Demux/1 -> Signal 1/1
  FromWs/1 -> Demux/1

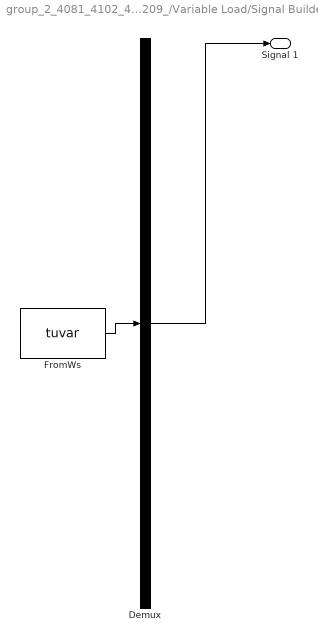
== system group_2_4081_4102_4209_/Variable Load/Signal Builder1 ==
  Demux : Demux  Tag=STV Demux  Outputs=1
      settings: DisplayOption=none
  FromWs : FromWorkspace  Tag=STV FromWs  VariableName=tuvar
      SigBuilderData=|
      | common.afterFinalStr = 'Extrapolate'
      | common.sampleTime = 0
      | dataSet.timeRange = [0 10]
      | dataSet.name = 'Group 1'
      | sbobj.Groups.Name = 'Group 1'
      | sbobj.Groups.Signals.Name = 'Signal 1'
      | sbobj.Groups.Signals.XData = [0 5 5 8 10]
      | sbobj.Groups.Signals.YData = [0 0 1 1 1]
  Signal 1 : Outport  Tag=STV Outport
  wires:
  Demux/1 -> Signal 1/1
  FromWs/1 -> Demux/1

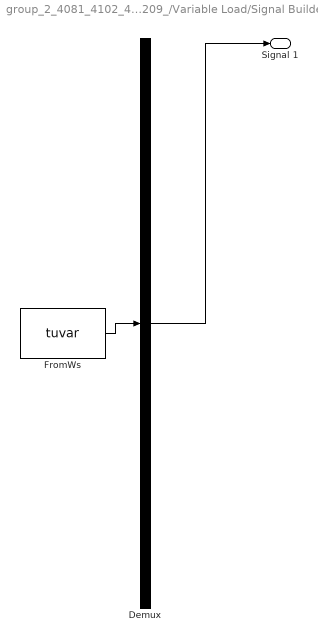
== system group_2_4081_4102_4209_/Variable Load/Signal Builder2 ==
  Demux : Demux  Tag=STV Demux  Outputs=1
      settings: DisplayOption=none
  FromWs : FromWorkspace  Tag=STV FromWs  VariableName=tuvar
      SigBuilderData=|
      | common.afterFinalStr = 'Extrapolate'
      | common.sampleTime = 0
      | dataSet.timeRange = [0 10]
      | dataSet.name = 'Group 1'
      | sbobj.Groups.Name = 'Group 1'
      | sbobj.Groups.Signals.Name = 'Signal 1'
      | sbobj.Groups.Signals.XData = [0 5 5 8 8 10]
      | sbobj.Groups.Signals.YData = [0 0 1 1 0 0]
  Signal 1 : Outport  Tag=STV Outport
  wires:
  Demux/1 -> Signal 1/1
  FromWs/1 -> Demux/1

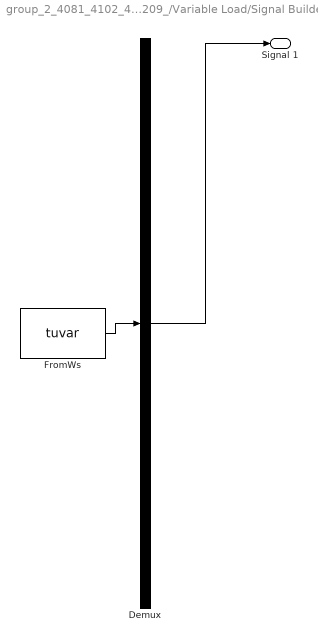
== system group_2_4081_4102_4209_/Variable Load/Signal Builder3 ==
  Demux : Demux  Tag=STV Demux  Outputs=1
      settings: DisplayOption=none
  FromWs : FromWorkspace  Tag=STV FromWs  VariableName=tuvar
      SigBuilderData=|
      | common.afterFinalStr = 'Extrapolate'
      | common.sampleTime = 0
      | dataSet.timeRange = [0 10]
      | dataSet.name = 'Group 1'
      | sbobj.Groups.Name = 'Group 1'
      | sbobj.Groups.Signals.Name = 'Signal 1'
      | sbobj.Groups.Signals.XData = [0 5 5 8 10]
      | sbobj.Groups.Signals.YData = [0 0 1 1 1]
  Signal 1 : Outport  Tag=STV Outport
  wires:
  Demux/1 -> Signal 1/1
  FromWs/1 -> Demux/1

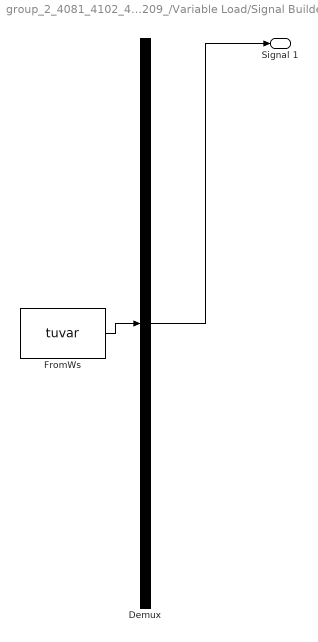
== system group_2_4081_4102_4209_/Variable Load/Signal Builder4 ==
  Demux : Demux  Tag=STV Demux  Outputs=1
      settings: DisplayOption=none
  FromWs : FromWorkspace  Tag=STV FromWs  VariableName=tuvar
      SigBuilderData=|
      | common.afterFinalStr = 'Extrapolate'
      | common.sampleTime = 0
      | dataSet.timeRange = [0 10]
      | dataSet.name = 'Group 1'
      | sbobj.Groups.Name = 'Group 1'
      | sbobj.Groups.Signals.Name = 'Signal 1'
      | sbobj.Groups.Signals.XData = [0 5 5 8 8 10]
      | sbobj.Groups.Signals.YData = [0 0 1 1 0 0]
  Signal 1 : Outport  Tag=STV Outport
  wires:
  Demux/1 -> Signal 1/1
  FromWs/1 -> Demux/1

== system group_2_4081_4102_4209_/Variable Load/Signal Builder5 ==
  Demux : Demux  Tag=STV Demux  Outputs=1
      settings: DisplayOption=none
  FromWs : FromWorkspace  Tag=STV FromWs  VariableName=tuvar
      SigBuilderData=|
      | common.afterFinalStr = 'Extrapolate'
      | common.sampleTime = 0
      | dataSet.timeRange = [0 10]
      | dataSet.name = 'Group 1'
      | sbobj.Groups.Name = 'Group 1'
      | sbobj.Groups.Signals.Name = 'Signal 1'
      | sbobj.Groups.Signals.XData = [0 5 5 8 10]
      | sbobj.Groups.Signals.YData = [0 0 1 1 1]
  Signal 1 : Outport  Tag=STV Outport
  wires:
  Demux/1 -> Signal 1/1
  FromWs/1 -> Demux/1

== matlab function group_2_4081_4102_4209_/MATLAB Function2 ==
  data: a input; result output; b input
function result = sqrtSumOfSquares(a, b)
% sqrtSumOfSquares - Returns the square root of the sum of the squares of two numbers
% Usage:
%   result = sqrtSumOfSquares(a, b)
%
% Inputs:
%   a - First input number
%   b - Second input number
%
% Output:
%   result - sqrt(a^2 + b^2)

    result = sqrt(a^2 + b^2);
end

== matlab function group_2_4081_4102_4209_/MATLAB Function3 ==
  data: a input; result output; b input
function result = sqrtSumOfSquares(a, b)
% sqrtSumOfSquares - Returns the square root of the sum of the squares of two numbers
% Usage:
%   result = sqrtSumOfSquares(a, b)
%
% Inputs:
%   a - First input number
%   b - Second input number
%
% Output:
%   result - sqrt(a^2 + b^2)

    result = sqrt(a^2 + b^2);
end

== matlab function group_2_4081_4102_4209_/MATLAB Function1 ==
  data: V input; duty output; I input; V_mpp output
function [duty, V_mpp] = incCondMPPT(V, I)

persistent V_prev I_prev duty_prev V_mpp_prev
alpha = 0.01;           % Step size for duty adjustment

% Initialize persistent variables
if isempty(V_prev)
    V_prev = V;
    I_prev = I;
    duty_prev = 0.5;      % Initial duty cycle
    V_mpp_prev = V;       % Initial MPP voltage
end

% Compute changes
dV = V - V_prev;
dI = I - I_prev;

% MPPT Logic
if dV == 0
    if dI == 0
        duty = duty_prev; % At MPP
        V_mpp = V_prev;
    elseif dI > 0
        duty = duty_prev - alpha;  % Increase voltage → Decrease duty
        V_mpp = V_prev;
    else
        duty = duty_prev + alpha;  % Decrease voltage → Increase duty
        V_mpp = V_prev;
    end
else
    IncCond = dI / dV;
    Cond = -I / V;

    if abs(IncCond - Cond) < 1e-4  % Close to MPP
        duty = duty_prev;
        V_mpp = V;                 % Save current voltage as MPP voltage
    elseif IncCond > Cond
        duty = duty_prev - alpha;  % Move toward MPP (left side)
        V_mpp = V_mpp_prev;
    else
        duty = duty_prev + alpha;  % Move toward MPP (right side)
        V_mpp = V_mpp_prev;
    end
end

% Clamp duty between 0 and 1
duty = max(0, min(1, duty));

% Update persistent variables
V_prev = V;
I_prev = I;
duty_prev = duty;

% Update stored MPP voltage only when very close to actual MPP
if abs(dI/dV + I/V) < 1e-4
    V_mpp_prev = V;
end

V_mpp = V_mpp_prev;

end
